simulink model "Final_Project"  (R2020a)
settings: Solver=FixedStepAuto  StartTime=0.0  StopTime=50  RelTol=1e-3  EnableMultiTasking=on
settings Model: SILPILModeSetting=veronly  ExtModeTrigDuration=2  Creator=s3864185  LastModifiedBy=doroke
settings OptimizationCC: EnhancedBackFolding=on  PassReuseOutputArgsAs=Individual arguments  ZeroExternalMemoryAtStartup=off  ZeroInternalMemoryAtStartup=off  MaxStackSize=64  OptimizeBlockOrder=speed  DifferentSizesBufferReuse=on  OptimizationCustomize=off  EfficientTunableParamExpr=on
settings DebuggingCC: ParameterTunabilityLossMsg=error
settings HardwareCC: ProdBitPerInt=16  ProdBitPerPointer=16  ProdBitPerSizeT=16  ProdBitPerPtrDiffT=16  ProdLargestAtomicFloat=None  ProdWordSize=8  ProdHWDeviceType=Atmel->AVR  UseEmbeddedCoderFeatures=off  UseSimulinkCoderFeatures=off
settings SFSimCC: MATLABDynamicMemAlloc=off
settings RTWCC: SystemTargetFile=ert.tlc  HardwareBoard=Arduino Uno  TLCOptions=-aInlineSetEventsForThisBaseRateFcn=TLC_FALSE -aSuppressMultiTaskScheduler=TLC_FALSE -aRateBasedStepFcn=1  TemplateMakefile=ert_default_tmf  Toolchain=Arduino AVR  BuildConfiguration=Faster Runs
settings CodeAppCC: ForceParamTrailComments=on  IgnoreCustomStorageClasses=off  OperatorAnnotations=on  SimulinkDataObjDesc=on  SFDataObjDesc=on  InsertBlockDesc=on
settings ERTTargetCC: SupportContinuousTime=on  SupportNonInlinedSFcns=on  SupportVariableSizeSignals=on  ExtModeStaticAllocSize=250

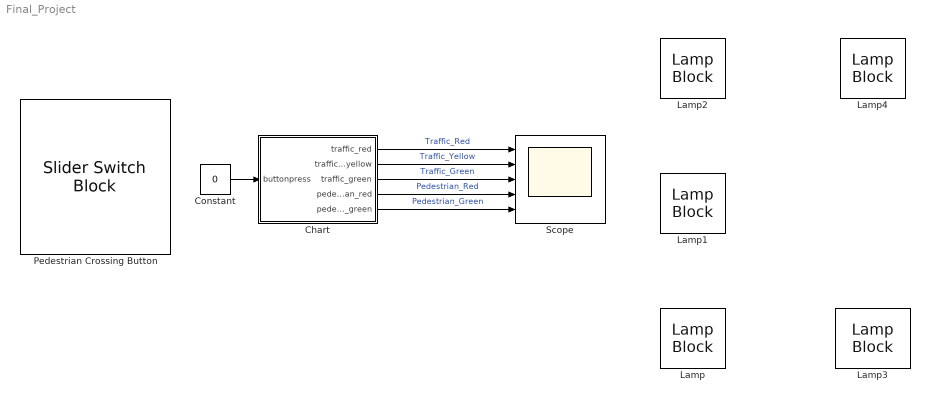
== system Final_Project ==
  Chart : Stateflow chart  TreatAsAtomicUnit=on
  Constant : Constant  Value=0
  Lamp{,1..4} (5 alike) : LampBlock
  Pedestrian Crossing Button : SliderSwitchBlock
      settings: Values={{'not pressed', 'pressed'}, [0 1]}
  Scope : Scope  NumInputPorts=5
  wires:
  Chart/1(traffic_red) -> Scope/1  "Traffic_Red"
  Chart/2(traffic_yellow) -> Scope/2  "Traffic_Yellow"
  Chart/3(traffic_green) -> Scope/3  "Traffic_Green"
  Chart/4(pedestrian_red) -> Scope/4  "Pedestrian_Red"
  Chart/5(pedestrian_green) -> Scope/5  "Pedestrian_Green"
  Constant/1 -> Chart/1(buttonpress)

== stateflow chart Final_Project/Chart ==
  state STATE1
    entry: traffic_red = 0;
    entry: traffic_yellow = 0;
    entry: traffic_green = 1;
    entry: pedestrian_red = 1;
    entry: pedestrian_green = 0;
  state STATE2
    entry: traffic_red = 0;
    entry: traffic_yellow = 1;
    entry: traffic_green = 0;
    entry: pedestrian_red = 1;
    entry: pedestrian_green = 0;
  state STATE3
    entry: traffic_red = 1;
    entry: traffic_yellow = 0;
    entry: traffic_green = 0;
    entry: pedestrian_red = 0;
    entry: pedestrian_green = 1;
  (default) -> STATE1
  STATE3 -> STATE1 : [after(6,sec)]
  STATE1 -> STATE2 : [buttonpress == 1]
  STATE2 -> STATE3 : [after(3,sec)]
  data: traffic_red output; traffic_yellow output; traffic_green output; pedestrian_red output; pedestrian_green output; buttonpress input
